simulink model "MPC_reduced"  (R2022a)
settings: Solver=VariableStepAuto  StartTime=0.0  StopTime=168  RelTol=1e-3
undefined symbols (not defined in the file): N, Ts, x0
libraries: mpclib x1
settings Model: Creator=tomok  LastModifiedBy=tomok

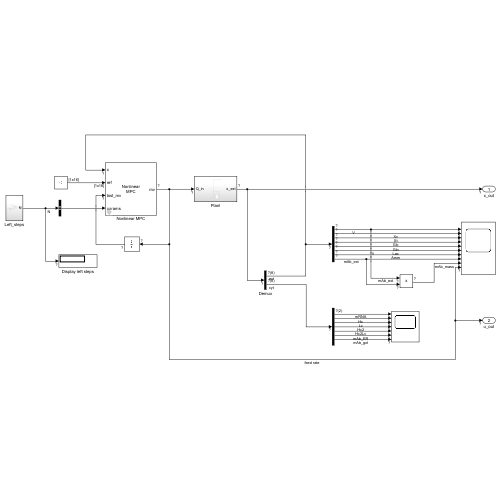
[thumbnail: Simulink's stored preview of the top-level diagram]
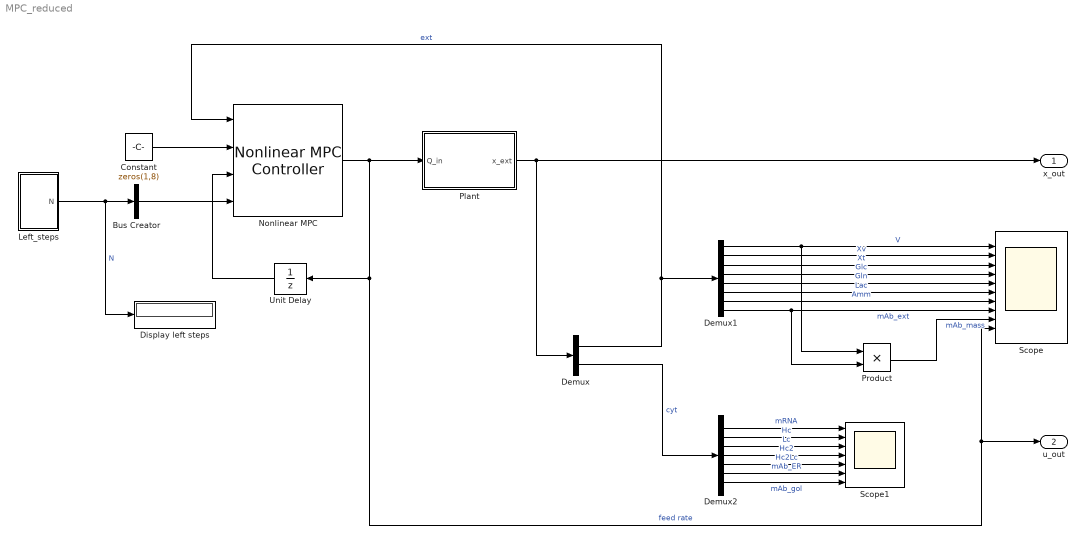
== system MPC_reduced ==
  Bus Creator : BusCreator  Inputs=1  OutDataTypeStr=Bus: myBusObject  NonVirtualBus=on
      settings: InheritFromInputs=off
  Constant : Constant  Value=zeros(1,8)  VectorParams1D=off
  Demux : Demux  Outputs=[8 8]
  Demux1 : Demux  Outputs=8
  Demux2 : Demux  Outputs=[2 1 1 1 1 1 1]
  Display left steps : Display
  Left_steps : Subsystem
  Nonlinear MPC : mpclib/Nonlinear MPC Controller  nlmpcobj=nlmpcReduced_error  UseObjectTs=on  UseMEX=off  md_enabled=off  mvtarget_enabled=off  param_enabled=on  cost_enabled=off  mvseq_enabled=off  stateseq_enabled=off  ovseq_enabled=off  slack_enabled=off  status_enabled=off  ov_min=off  ov_max=off  mv_min=off  mv_max=off  mvrate_min=off  mvrate_max=off  state_min=off  state_max=off  ov_weight=off  mv_weight=off  mvrate_weight=off  ecr_weight=off  nlp_initialize=off
  Plant : Subsystem
  Product : Product
  Scope : Scope  NumInputPorts=10
  Scope1 : Scope  NumInputPorts=7
  Unit Delay : UnitDelay  SampleTime=-1  HasFrameUpgradeWarning=on
  x_out : Outport
  u_out : Outport  Port=2
  wires:
  Nonlinear MPC/1 -> Scope/10, u_out/1, Unit Delay/1, Plant/1(Q_in)  "feed rate"
  Constant/1 -> Nonlinear MPC/2
  Unit Delay/1 -> Nonlinear MPC/3
  Bus Creator/1 -> Nonlinear MPC/4
  Left_steps/1(N) -> Display left steps/1, Bus Creator/1  "N"
  Plant/1(x_ext) -> x_out/1, Demux/1
  Product/1 -> Scope/9  "mAb_mass"
  Demux2/4 -> Scope1/4  "Hc2"
  Demux/2 -> Demux2/1  "cyt"
  Demux2/2 -> Scope1/2  "Hc"
  Demux2/6 -> Scope1/6  "mAb_ER"
  Demux1/4 -> Scope/4  "Glc"
  Demux2/3 -> Scope1/3  "Lc"
  Demux1/8 -> Product/2, Scope/8  "mAb_ext"
  Demux1/1 -> Product/1, Scope/1  "V"
  Demux1/5 -> Scope/5  "Gln"
  Demux1/3 -> Scope/3  "Xt"
  Demux2/1 -> Scope1/1  "mRNA"
  Demux/1 -> Nonlinear MPC/1, Demux1/1  "ext"
  Demux2/7 -> Scope1/7  "mAb_gol"
  Demux1/6 -> Scope/6  "Lac"
  Demux1/7 -> Scope/7  "Amm"
  Demux2/5 -> Scope1/5  "Hc2Lc"
  Demux1/2 -> Scope/2  "Xv"

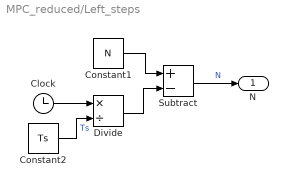
== system MPC_reduced/Left_steps ==
  Clock : Clock
  Constant1 : Constant  Value=N
  Constant2 : Constant  Value=Ts
  Divide : Product  Inputs=*/
  Subtract : Sum  Inputs=+-
  N : Outport
  wires:
  Constant2/1 -> Divide/2  "Ts"
  Divide/1 -> Subtract/2
  Clock/1 -> Divide/1
  Subtract/1 -> N/1  "N"
  Constant1/1 -> Subtract/1

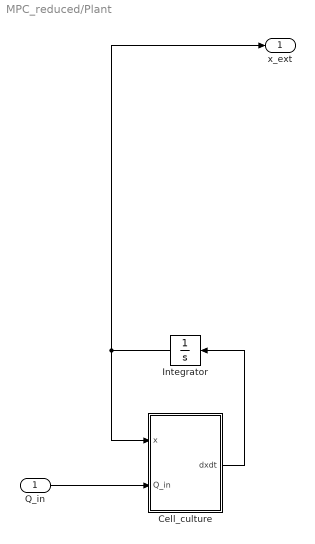
== system MPC_reduced/Plant ==
  Q_in : Inport
  Cell_culture : MATLAB Function  TreatAsAtomicUnit=on
  Integrator : Integrator  InitialCondition=x0  LimitOutput=on  LowerSaturationLimit=0
  x_ext : Outport
  wires:
  Cell_culture/1(dxdt) -> Integrator/1
  Q_in/1 -> Cell_culture/2(Q_in)
  Integrator/1 -> x_ext/1, Cell_culture/1(x)

== matlab function MPC_reduced/Plant/Cell_culture ==
  data: dxdt output; x input; Q_in input
function dxdt = fcn(x,Q_in)
dxdt = Kontoravdi2010StateFcn(x,Q_in);
end
